simulink model "group2_assignment2_pacemaker"  (R2023b)
settings: Solver=FixedStepAuto  StartTime=0.0  StopTime=10  FixedStep=1e-3  RelTol=1e-3  EnableMultiTasking=on
undefined symbols (not defined in the file): D0, D1, D10, D11, D12, D13, D2, D3, D4, D5, D6, D7, D8, D9, PTA0, PTA1, PTA2, PTB23, PTB9, PTC16, PTC17, PTC2, PTC3, PTC4, PTD0, PTD1, PTD2, PTD3
libraries: frdmk64flib x15, dspstat3 x1
settings Model: SimulationMode=external  ExtModeTrigDuration=5  Creator=stivb  LastModifiedBy=conno
settings OptimizationCC: EnhancedBackFolding=on  PassReuseOutputArgsAs=Individual arguments  ZeroExternalMemoryAtStartup=off  ZeroInternalMemoryAtStartup=off  MaxStackSize=64  OptimizeBlockOrder=speed  DifferentSizesBufferReuse=on  OptimizationCustomize=off  EfficientTunableParamExpr=on
settings DebuggingCC: ParameterTunabilityLossMsg=error
settings HardwareCC: ProdBitPerPointer=32  ProdBitPerSizeT=32  ProdBitPerPtrDiffT=32  ProdLargestAtomicInteger=Long  ProdLargestAtomicFloat=Double  ProdWordSize=32  ProdHWDeviceType=ARM Compatible->ARM Cortex
settings RTWCC: Description=Embedded Coder  SystemTargetFile=ert.tlc  HardwareBoard=NXP FRDM-K64F  TLCOptions="-aInlineSetEventsForThisBaseRateFcn=TLC_FALSE -aSuppressMultiTaskScheduler=TLC_FALSE  -aRateBasedStepFcn=0"  TemplateMakefile=ert_default_tmf  Toolchain=GNU Tools for ARM Embedded Processors
settings CodeAppCC: ForceParamTrailComments=on  IgnoreCustomStorageClasses=off  OperatorAnnotations=on  SimulinkDataObjDesc=on  SFDataObjDesc=on  InsertBlockDesc=on
settings ERTTargetCC: SupportContinuousTime=on  SupportVariableSizeSignals=on  ExtMode=on  ExtModeTransport=4  ExtModeMexFile=sendToCommService  ExtModeMexArgs='group2_assignment2_pacemaker' 0

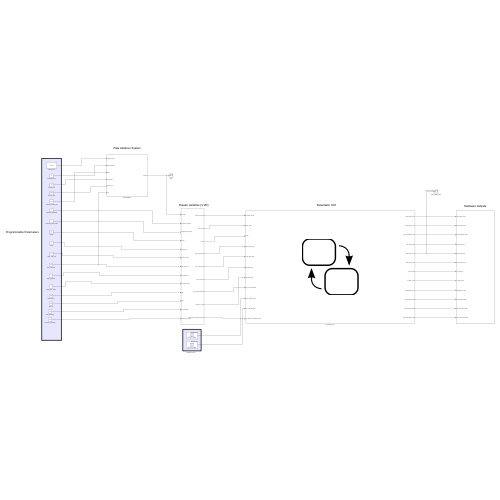
[thumbnail: Simulink's stored preview of the top-level diagram]
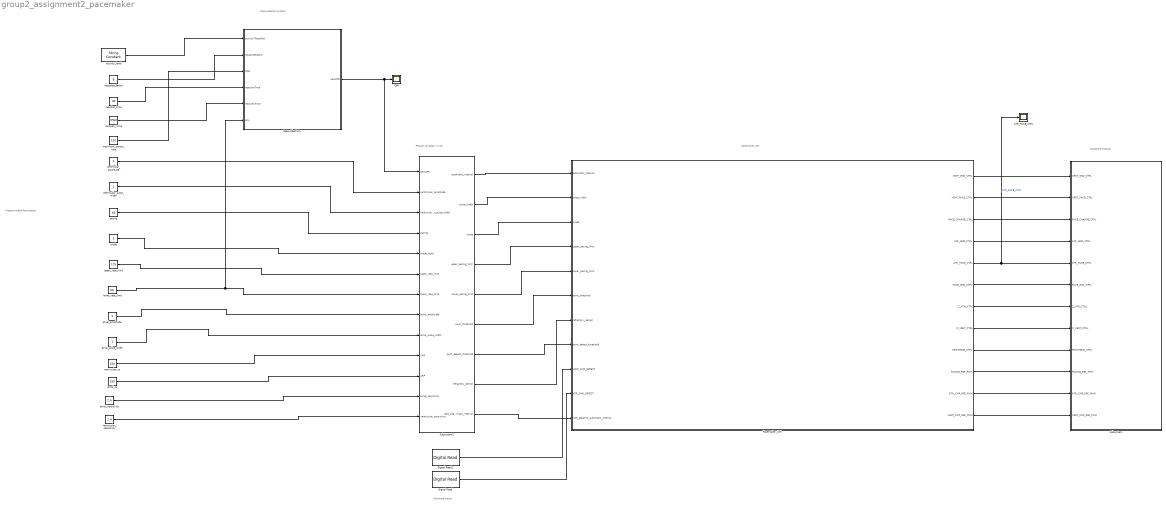
== system group2_assignment2_pacemaker ==
  note: Rate Adaption System
  note: Hardware inputs
  note: Pseudo variables (4 VM)
  note: Programmable Parameters
  note: Pacemaker Unit
  note: Hardware Outputs
  ATR_PACE_CTRL : Scope
  CPR : Scope
  Digital Read : frdmk64flib/Digital Read  Whichpin=PTC16 (D0)  SampleTime=-1
  Digital Read1 : frdmk64flib/Digital Read  Whichpin=PTC17 (D1)  SampleTime=-1
  Pacemaker_Unit : Stateflow chart  TreatAsAtomicUnit=on
      settings: PortSchema="{\"entries\":[{\"content\":{\"sides\":[{\"content\":{\"connectorIds\":[\"In1\",\"In2\",\"In4\",\"In3\",\"In5\",\"In6\",\"In7\",\"In8\",\"In10\",\"In9\",\"In11\"]},\"type\":\"ConnectorPlacement.EquallySpacedRectSide\",\"uuid\":\"c8cba9b3-707c-4f69-ad8c-9d5fbaa12caa\"},{\"content\":{\"connectorIds\":[\"Out1\",\"Out2\",\"Out3\",\"Out4\",\"Out5\",\"Out6\",\"Out7\",\"Out8\",\"Out9\",\"Out10\",\"Out11\",\"Out12\"],\"side\":\"RIGHT\"},\"type\":\"ConnectorPlacement.EquallySpacedRectSide\",\"uuid\":\"918aa1e0-aae1-41d7-a74d-0a72155b1f75\"},{\"content\":{\"side\":\"TOP\"},\"type\":\"ConnectorPlacement.EquallySpacedRectSide\",\"uuid\":\"877803b3-29d8-4e86-807a-7bf9f59cc519\"}]},\"type\":\"ConnectorPlacement.EquallySpacedConnector\",\"uuid\":\"1e148aae-cf3c-4ae1-bc6b-9e679c8c5f2a\"}],\"packageUris\":[\"http://schema.mathworks.com/mf0/Connector/R2020b\"],\"version\":\"1.0\"}"
  Rate Adaptivity : Subsystem
  Subsystem : Subsystem
  Subsystem2 : Subsystem
  activity_level : StringConstant  String="\"V-Low\""
  atrial_amplitude : Constant
  atrial_pulse_width : Constant
  atrial_rp : Constant  Value=150
  atrial_sensitivity : Constant  Value=2.4
  lower_rate_limit : Constant  Value=60
  maximum_sensor_rate : Constant  Value=120
  mode : Constant  Value=3
  pacing : Constant  Value=60
  reaction_time : Constant  Value=30
  recovery_time : Constant  Value=5*60
  response_factor : Constant  Value=8
  upper_rate_limit : Constant  Value=175
  ventricular_amplitude : Constant  Value=4
  ventricular_pulse_width : Constant
  ventricular_rp : Constant  Value=150
  ventricular_sensitivity : Constant  Value=2.4
  wires:
  mode/1 -> Subsystem2/5(mode_input)
  ventricular_amplitude/1 -> Subsystem2/2(ventricular_amplitude)
  atrial_amplitude/1 -> Subsystem2/8(atrial_amplitude)
  atrial_pulse_width/1 -> Subsystem2/9(atrial_pulse_width)
  lower_rate_limit/1 -> Rate Adaptivity/6(LRL), Subsystem2/7(lower_rate_limit)
  upper_rate_limit/1 -> Subsystem2/6(upper_rate_limit)
  ventricular_pulse_width/1 -> Subsystem2/3(ventricular_pulse_width)
  pacing/1 -> Subsystem2/4(pacing)
  Subsystem2/1(automatic_interval) -> Pacemaker_Unit/1(automatic_interval)
  Subsystem2/2(pulse_width) -> Pacemaker_Unit/2(pulse_width)
  Subsystem2/3(mode) -> Pacemaker_Unit/4(mode)
  Subsystem2/4(upper_pacing_limit) -> Pacemaker_Unit/3(upper_pacing_limit)
  Subsystem2/5(lower_pacing_limit) -> Pacemaker_Unit/5(lower_pacing_limit)
  Subsystem2/6(pwm_threshold) -> Pacemaker_Unit/6(pwm_threshold)
  Subsystem2/8(refractory_period) -> Pacemaker_Unit/7(refractory_period)
  Pacemaker_Unit/1(VENT_GND_CTRL) -> Subsystem/1(VENT_GND_CTRL)
  Pacemaker_Unit/2(VENT_PACE_CTRL) -> Subsystem/2(VENT_PACE_CTRL)
  Pacemaker_Unit/3(PACE_CHARGE_CTRL) -> Subsystem/3(PACE_CHARGE_CTRL)
  Pacemaker_Unit/4(ATR_GND_CTRL) -> Subsystem/4(ATR_GND_CTRL)
  Pacemaker_Unit/5(ATR_PACE_CTRL) -> ATR_PACE_CTRL/1, Subsystem/5(ATR_PACE_CTRL)  "ATR_PACE_CTRL"
  Pacemaker_Unit/6(PACE_GND_CTRL) -> Subsystem/6(PACE_GND_CTRL)
  Pacemaker_Unit/7(Z_ATR_CTRL) -> Subsystem/7(Z_ATR_CTRL)
  Pacemaker_Unit/8(Z_VENT_CTRL) -> Subsystem/8(Z_VENT_CTRL)
  Pacemaker_Unit/9(FRONTEND_CTRL) -> Subsystem/9(FRONTEND_CTRL)
  Pacemaker_Unit/10(PACING_REF_PWM) -> Subsystem/10(PACING_REF_PWM)
  ventricular_rp/1 -> Subsystem2/10(VRP)
  atrial_rp/1 -> Subsystem2/11(ARP)
  Pacemaker_Unit/11(ATR_CMP_REF_PWM) -> Subsystem/11(ATR_CMP_REF_PWM)
  Digital Read/1 -> Pacemaker_Unit/9(ATR_CMP_DETECT)
  Digital Read1/1 -> Pacemaker_Unit/10(VENT_CMP_DETECT)
  atrial_sensitivity/1 -> Subsystem2/12(atrial_sensitivity)
  ventricular_sensitivity/1 -> Subsystem2/13(ventricular_sensitivity)
  Subsystem2/7(pwm_detect_threshold) -> Pacemaker_Unit/8(pwm_detect_threshold)
  Pacemaker_Unit/12(VENT_CMP_REF_PWM) -> Subsystem/12(VENT_CMP_REF_PWM)
  Subsystem2/9(rate_adaptive_automatic_interval) -> Pacemaker_Unit/11(rate_adaptive_automatic_interval)
  activity_level/1 -> Rate Adaptivity/1(activityThreshold)
  response_factor/1 -> Rate Adaptivity/2(responseFactor)
  maximum_sensor_rate/1 -> Rate Adaptivity/3(MSR)
  reaction_time/1 -> Rate Adaptivity/4(reactionTime)
  recovery_time/1 -> Rate Adaptivity/5(recoveryTime)
  Rate Adaptivity/1(newCPR) -> CPR/1, Subsystem2/1(newCPR)

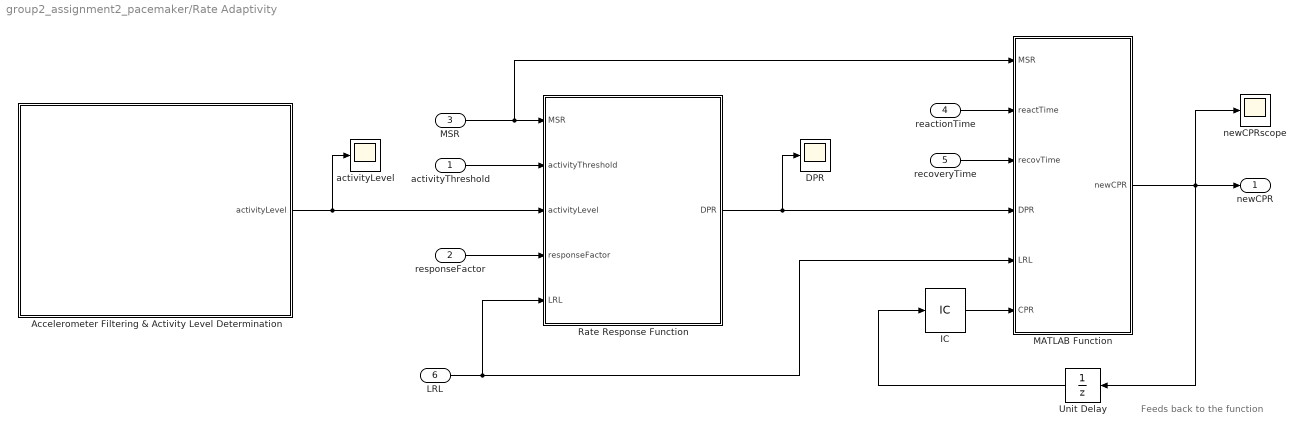
== system group2_assignment2_pacemaker/Rate Adaptivity ==
  note: Feeds back to the function
  activityThreshold : Inport
  responseFactor : Inport  Port=2
  MSR : Inport  Port=3
  reactionTime : Inport  Port=4
  recoveryTime : Inport  Port=5
  LRL : Inport  Port=6
  Accelerometer Filtering & Activity Level Determination : Subsystem
  DPR : Scope
  IC : InitialCondition  Value=80
  MATLAB Function : MATLAB Function  TreatAsAtomicUnit=on
  Rate Response Function : MATLAB Function  TreatAsAtomicUnit=on
  Unit Delay : UnitDelay  SampleTime=-1  HasFrameUpgradeWarning=on
  activityLevel : Scope
  newCPRscope : Scope
  newCPR : Outport
  wires:
  LRL/1 -> MATLAB Function/5(LRL), Rate Response Function/5(LRL)
  activityThreshold/1 -> Rate Response Function/2(activityThreshold)
  MSR/1 -> MATLAB Function/1(MSR), Rate Response Function/1(MSR)
  responseFactor/1 -> Rate Response Function/4(responseFactor)
  recoveryTime/1 -> MATLAB Function/3(recovTime)
  MATLAB Function/1(newCPR) -> Unit Delay/1, newCPR/1, newCPRscope/1
  reactionTime/1 -> MATLAB Function/2(reactTime)
  Rate Response Function/1(DPR) -> MATLAB Function/4(DPR), DPR/1
  Unit Delay/1 -> IC/1
  IC/1 -> MATLAB Function/6(CPR)
  Accelerometer Filtering & Activity Level Determination/1(activityLevel) -> Rate Response Function/3(activityLevel), activityLevel/1

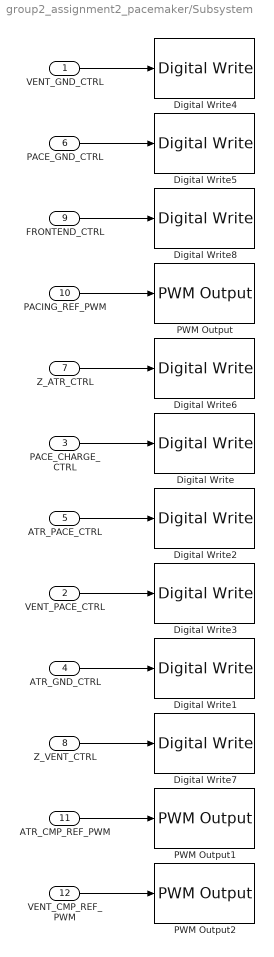
== system group2_assignment2_pacemaker/Subsystem ==
  VENT_GND_CTRL : Inport
  VENT_PACE_CTRL : Inport  Port=2
  PACE_CHARGE_CTRL : Inport  Port=3
  ATR_GND_CTRL : Inport  Port=4
  ATR_PACE_CTRL : Inport  Port=5
  PACE_GND_CTRL : Inport  Port=6
  Z_ATR_CTRL : Inport  Port=7
  Z_VENT_CTRL : Inport  Port=8
  FRONTEND_CTRL : Inport  Port=9
  PACING_REF_PWM : Inport  Port=10
  ATR_CMP_REF_PWM : Inport  Port=11
  VENT_CMP_REF_PWM : Inport  Port=12
  Digital Write : frdmk64flib/Digital Write  Whichpin=PTB9 (D2)
  Digital Write1 : frdmk64flib/Digital Write  Whichpin=PTD2 (D11)
  Digital Write2 : frdmk64flib/Digital Write  Whichpin=PTA0 (D8)
  Digital Write3 : frdmk64flib/Digital Write  Whichpin=PTC4 (D9)
  Digital Write4 : frdmk64flib/Digital Write  Whichpin=PTD3 (D12)
  Digital Write5 : frdmk64flib/Digital Write  Whichpin=PTD0 (D10)
  Digital Write6 : frdmk64flib/Digital Write  Whichpin=PTB23 (D4)
  Digital Write7 : frdmk64flib/Digital Write  Whichpin=PTC3 (D7)
  Digital Write8 : frdmk64flib/Digital Write  Whichpin=PTD1 (D13)
  PWM Output : frdmk64flib/PWM Output  Whichpin=PTA2 (D5)  InitialFrequency=2000  InitialDutyCycle=0
  PWM Output1 : frdmk64flib/PWM Output  Whichpin=PTC2 (D6)  InitialFrequency=2000  InitialDutyCycle=0
  PWM Output2 : frdmk64flib/PWM Output  Whichpin=PTA1 (D3)  InitialFrequency=2000  InitialDutyCycle=0
  wires:
  Z_ATR_CTRL/1 -> Digital Write6/1
  VENT_PACE_CTRL/1 -> Digital Write3/1
  FRONTEND_CTRL/1 -> Digital Write8/1
  PACING_REF_PWM/1 -> PWM Output/1
  ATR_PACE_CTRL/1 -> Digital Write2/1
  Z_VENT_CTRL/1 -> Digital Write7/1
  VENT_GND_CTRL/1 -> Digital Write4/1
  PACE_CHARGE_CTRL/1 -> Digital Write/1
  ATR_GND_CTRL/1 -> Digital Write1/1
  PACE_GND_CTRL/1 -> Digital Write5/1
  ATR_CMP_REF_PWM/1 -> PWM Output1/1
  VENT_CMP_REF_PWM/1 -> PWM Output2/1

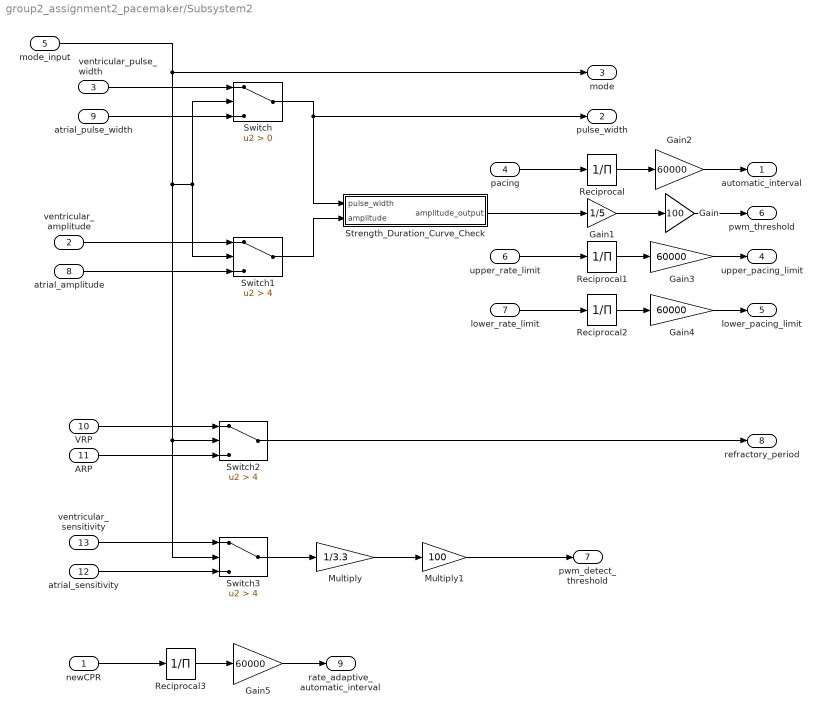
== system group2_assignment2_pacemaker/Subsystem2 ==
  newCPR : Inport
  ventricular_amplitude : Inport  Port=2
  ventricular_pulse_width : Inport  Port=3
  pacing : Inport  Port=4
  mode_input : Inport  Port=5
  upper_rate_limit : Inport  Port=6
  lower_rate_limit : Inport  Port=7
  atrial_amplitude : Inport  Port=8
  atrial_pulse_width : Inport  Port=9
  VRP : Inport  Port=10
  ARP : Inport  Port=11
  atrial_sensitivity : Inport  Port=12
  ventricular_sensitivity : Inport  Port=13
  Gain : Gain  Gain=100
  Gain1 : Gain  Gain=1/5
  Gain{2..5} (4 alike) : Gain  Gain=60000
  Multiply : Gain  Gain=1/3.3
  Multiply1 : Gain  Gain=100
  Reciprocal{,1..3} (4 alike) : Product  Inputs=/
  Strength_Duration_Curve_Check : Stateflow chart  TreatAsAtomicUnit=on
  Switch : Switch  Criteria=u2 > Threshold  SaturateOnIntegerOverflow=off  InputSameDT=off
  Switch1 : Switch  Criteria=u2 > Threshold  Threshold=4  SaturateOnIntegerOverflow=off  InputSameDT=off
  Switch2 : Switch  Criteria=u2 > Threshold  Threshold=4  SaturateOnIntegerOverflow=off  InputSameDT=off
  Switch3 : Switch  Criteria=u2 > Threshold  Threshold=4  SaturateOnIntegerOverflow=off  InputSameDT=off
  automatic_interval : Outport
  pulse_width : Outport  Port=2
  mode : Outport  Port=3
  upper_pacing_limit : Outport  Port=4
  lower_pacing_limit : Outport  Port=5
  pwm_threshold : Outport  Port=6
  pwm_detect_threshold : Outport  Port=7
  refractory_period : Outport  Port=8
  rate_adaptive_automatic_interval : Outport  Port=9
  wires:
  Gain1/1 -> Gain/1
  pacing/1 -> Reciprocal/1
  Reciprocal1/1 -> Gain3/1
  upper_rate_limit/1 -> Reciprocal1/1
  Reciprocal/1 -> Gain2/1
  Gain2/1 -> automatic_interval/1
  Gain/1 -> pwm_threshold/1
  Gain3/1 -> upper_pacing_limit/1
  Strength_Duration_Curve_Check/1(amplitude_output) -> Gain1/1
  Reciprocal2/1 -> Gain4/1
  lower_rate_limit/1 -> Reciprocal2/1
  Gain4/1 -> lower_pacing_limit/1
  Switch1/1 -> Strength_Duration_Curve_Check/2(amplitude)
  Switch/1 -> Strength_Duration_Curve_Check/1(pulse_width), pulse_width/1
  Switch2/1 -> refractory_period/1
  VRP/1 -> Switch2/1
  ARP/1 -> Switch2/3
  ventricular_amplitude/1 -> Switch1/1
  ventricular_pulse_width/1 -> Switch/1
  atrial_pulse_width/1 -> Switch/3
  atrial_amplitude/1 -> Switch1/3
  mode_input/1 -> Switch3/2, Switch2/2, Switch1/2, Switch/2, mode/1
  atrial_sensitivity/1 -> Switch3/3
  ventricular_sensitivity/1 -> Switch3/1
  Switch3/1 -> Multiply/1
  Multiply/1 -> Multiply1/1
  Multiply1/1 -> pwm_detect_threshold/1
  Gain5/1 -> rate_adaptive_automatic_interval/1
  Reciprocal3/1 -> Gain5/1
  newCPR/1 -> Reciprocal3/1

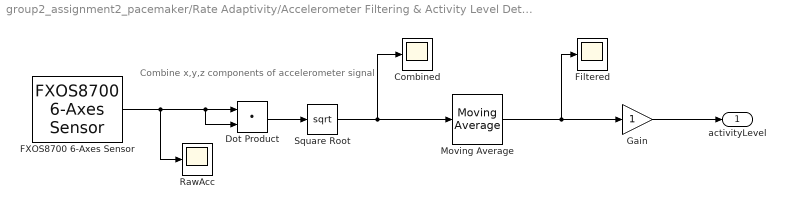
== system group2_assignment2_pacemaker/Rate Adaptivity/Accelerometer Filtering & Activity Level Determination ==
  note: Combine x,y,z components of accelerometer signal
  Combined : Scope
  Dot Product : DotProduct  OutDataTypeStr=Inherit: Inherit via internal rule
  FXOS8700 6-Axes Sensor : frdmk64flib/FXOS8700 6-Axes Sensor  Activesensor=Accelerometer only  ODR=800Hz  HybridODR=400Hz  Accelfullrange=-4g to +4g  SampleTime=-1
  Filtered : Scope
  Gain : Gain
  Moving Average : dspstat3/Moving Average  Method=Sliding window  ForgettingFactorPort=off  SpecifyWindowLength=on  WindowLength=4  OverlapLength=3  AllowArbitraryInputLength=off  ForgettingFactor=0.9  SimulateUsing=Code generation
  RawAcc : Scope
  Square Root : Sqrt
  activityLevel : Outport
  wires:
  Moving Average/1 -> Filtered/1, Gain/1
  Square Root/1 -> Moving Average/1, Combined/1
  Dot Product/1 -> Square Root/1
  FXOS8700 6-Axes Sensor/1 -> Dot Product/1, Dot Product/2, RawAcc/1
  Gain/1 -> activityLevel/1

== stateflow chart group2_assignment2_pacemaker/Pacemaker_Unit ==
  state VOO
    state Charge_C22_Discharge_C21
      entry:
      %Charge C22
      VENT_PACE_CTRL = 0;
      PACE_CHARGE_CTRL = 1;
      %Discharge C21
      VENT_GND_CTRL= 1;
    state ChargeC21_and_DischargeC22
      %Creates the leading edge and sends pulse for X amount of time
      entry:
      PACE_CHARGE_CTRL = 0;
      VENT_GND_CTRL = 0;
      VENT_PACE_CTRL = 1;
      %Recharge pulse is the current in the opposite direction due to C21
    (default) -> VOO.Charge_C22_Discharge_C21
    VOO.Charge_C22_Discharge_C21 -> VOO.ChargeC21_and_DischargeC22 : after(automatic_interval-pulse_width, msec)
    VOO.ChargeC21_and_DischargeC22 -> VOO.Charge_C22_Discharge_C21 : after(pulse_width, msec)
  state VVI
    note: Safe start entry; since hysteresis pacing allows for waiting a period of time longer than the refractory period, we are okay with waiting a refractory period of time before we start pacing. This also ensures that the capacitors are appropriately charged to allow for proper pacing.
    state Refractory_and_charging_ventricle
      entry:
      %Charge C22
      VENT_PACE_CTRL = 0;
      PACE_CHARGE_CTRL = 1;
      %Discharge C21
      VENT_GND_CTRL= 1;
      % Setup sensing pins
      VENT_CMP_REF_PWM = pwm_detect_threshold;
    note: Detected a pace, so go back to refractory state to wait
        | the appropriate refractory time interval
    state Sensing_ventricle
      entry:
      FRONTEND_CTRL = 1;
    state Pacing_ventricle
      entry:
      PACE_CHARGE_CTRL = 0;
      VENT_PACE_CTRL = 1;
      VENT_GND_CTRL = 0;
    (default) -> VVI.Refractory_and_charging_ventricle
    VVI.Refractory_and_charging_ventricle -> VVI.Sensing_ventricle : after(refractory_period, msec)
    VVI.Sensing_ventricle -> VVI.Refractory_and_charging_ventricle [order 1] : [VENT_CMP_DETECT == true]
    VVI.Pacing_ventricle -> VVI.Refractory_and_charging_ventricle : after(pulse_width, msec)
    VVI.Sensing_ventricle -> VVI.Pacing_ventricle [order 2] : after(automatic_interval - refractory_period - pulse_width, msec)
  state Ventricular_Safe_State
    entry: %Safe State
    ATR_PACE_CTRL = 0;
    VENT_PACE_CTRL=0;
    PACING_REF_PWM = pwm_threshold;
    PACE_CHARGE_CTRL=0;
    PACE_GND_CTRL = 1;
    VENT_PACE_CTRL=0;
    Z_ATR_CTRL=0;
    Z_VENT_CTRL=0;
    ATR_PACE_CTRL=0;
    ATR_GND_CTRL=0;
    VENT_GND_CTRL=1;
    FRONTEND_CTRL=0;
  state VOOR
    state Charge_C22_Discharge_C21
      entry:
      %Charge C22
      VENT_PACE_CTRL = 0;
      PACE_CHARGE_CTRL = 1;
      %Discharge C21
      VENT_GND_CTRL= 1;
    state ChargeC21_and_DischargeC22
      %Creates the leading edge and sends pulse for X amount of time
      entry:
      PACE_CHARGE_CTRL = 0;
      VENT_GND_CTRL = 0;
      VENT_PACE_CTRL = 1;
      %Recharge pulse is the current in the opposite direction due to C21
    (default) -> VOOR.Charge_C22_Discharge_C21
    VOOR.Charge_C22_Discharge_C21 -> VOOR.ChargeC21_and_DischargeC22 : after(rate_adaptive_automatic_interval-pulse_width, msec)
    VOOR.ChargeC21_and_DischargeC22 -> VOOR.Charge_C22_Discharge_C21 : after(pulse_width, msec)
  state VVIR
    note: Safe start entry; since hysteresis pacing allows for waiting a period of time longer than the refractory period, we are okay with waiting a refractory period of time before we start pacing. This also ensures that the capacitors are appropriately charged to allow for proper pacing.
    state Refractory_and_charging_ventricle
      entry:
      %Charge C22
      VENT_PACE_CTRL = 0;
      PACE_CHARGE_CTRL = 1;
      %Discharge C21
      VENT_GND_CTRL= 1;
      % Setup sensing pins
      VENT_CMP_REF_PWM = pwm_detect_threshold;
    note: Detected a pace, so go back to refractory state to wait
        | the appropriate refractory time interval
    state Sensing_ventricle
      entry:
      FRONTEND_CTRL = 1;
    state Pacing_ventricle
      entry:
      PACE_CHARGE_CTRL = 0;
      VENT_PACE_CTRL = 1;
      VENT_GND_CTRL = 0;
    (default) -> VVIR.Refractory_and_charging_ventricle
    VVIR.Refractory_and_charging_ventricle -> VVIR.Sensing_ventricle : after(refractory_period, msec)
    VVIR.Sensing_ventricle -> VVIR.Refractory_and_charging_ventricle [order 1] : [VENT_CMP_DETECT == true]
    VVIR.Pacing_ventricle -> VVIR.Refractory_and_charging_ventricle : after(pulse_width, msec)
    VVIR.Sensing_ventricle -> VVIR.Pacing_ventricle [order 2] : after(rate_adaptive_automatic_interval - refractory_period - pulse_width, msec)
  state Mode_Selection
  state AAIR
    note: Safe start entry; since hysteresis pacing allows for waiting a period of time longer than the refractory period, we are okay with waiting a refractory period of time before we start pacing. This also ensures that the capacitors are appropriately charged to allow for proper pacing.
    state Refractory_and_charging_atrial
      entry:
      %Charge C22
      ATR_PACE_CTRL = 0;
      PACE_CHARGE_CTRL = 1;
      %Discharge C21
      ATR_GND_CTRL= 1;
      % Setup sensing pins
      ATR_CMP_REF_PWM = pwm_detect_threshold;
    note: Detected a pace, so go back to refractory state to wait
        | the appropriate refractory time interval
    state Sensing_atrial
      entry:
      FRONTEND_CTRL = 1;
    state Pacing_atrial
      entry:
      PACE_CHARGE_CTRL = 0;
      ATR_PACE_CTRL = 1;
      ATR_GND_CTRL = 0;
    (default) -> AAIR.Refractory_and_charging_atrial
    AAIR.Refractory_and_charging_atrial -> AAIR.Sensing_atrial : after(refractory_period, msec)
    AAIR.Sensing_atrial -> AAIR.Refractory_and_charging_atrial [order 1] : [ATR_CMP_DETECT == true]
    AAIR.Pacing_atrial -> AAIR.Refractory_and_charging_atrial : after(pulse_width, msec)
    AAIR.Sensing_atrial -> AAIR.Pacing_atrial [order 2] : after(rate_adaptive_automatic_interval - refractory_period - pulse_width, msec)
  state Atrial_Safe_State
    entry: %Safe State
    ATR_PACE_CTRL = 0;
    VENT_PACE_CTRL=0;
    PACING_REF_PWM = pwm_threshold;
    PACE_CHARGE_CTRL=0;
    PACE_GND_CTRL = 1;
    VENT_PACE_CTRL=0;
    Z_ATR_CTRL=0;
    Z_VENT_CTRL=0;
    ATR_PACE_CTRL=0;
    ATR_GND_CTRL=1;
    VENT_GND_CTRL=0;
    FRONTEND_CTRL=0;
  state AOOR
    state Charge_C22_Discharge_C21
      entry:
      %Charge C22
      ATR_PACE_CTRL = 0;
      PACE_CHARGE_CTRL = 1;
      %Discharge C21
      ATR_GND_CTRL= 1;
    state ChargeC21_and_DischargeC22
      %Creates the leading edge and sends pulse for X amount of time
      entry:
      PACE_CHARGE_CTRL = 0;
      ATR_PACE_CTRL = 1;
      ATR_GND_CTRL = 0;
    (default) -> AOOR.Charge_C22_Discharge_C21
    AOOR.Charge_C22_Discharge_C21 -> AOOR.ChargeC21_and_DischargeC22 : after(rate_adaptive_automatic_interval-pulse_width, msec)
    AOOR.ChargeC21_and_DischargeC22 -> AOOR.Charge_C22_Discharge_C21 : after(pulse_width, msec)
  state AAI
    note: Safe start entry; since hysteresis pacing allows for waiting a period of time longer than the refractory period, we are okay with waiting a refractory period of time before we start pacing. This also ensures that the capacitors are appropriately charged to allow for proper pacing.
    state Refractory_and_charging_atrial
      entry:
      %Charge C22
      ATR_PACE_CTRL = 0;
      PACE_CHARGE_CTRL = 1;
      %Discharge C21
      ATR_GND_CTRL= 1;
      % Setup sensing pins
      ATR_CMP_REF_PWM = pwm_detect_threshold;
    note: Detected a pace, so go back to refractory state to wait
        | the appropriate refractory time interval
    state Sensing_atrial
      entry:
      FRONTEND_CTRL = 1;
    state Pacing_atrial
      entry:
      PACE_CHARGE_CTRL = 0;
      ATR_PACE_CTRL = 1;
      ATR_GND_CTRL = 0;
    (default) -> AAI.Refractory_and_charging_atrial
    AAI.Refractory_and_charging_atrial -> AAI.Sensing_atrial : after(refractory_period, msec)
    AAI.Sensing_atrial -> AAI.Refractory_and_charging_atrial [order 1] : [ATR_CMP_DETECT == true]
    AAI.Pacing_atrial -> AAI.Refractory_and_charging_atrial : after(pulse_width, msec)
    AAI.Sensing_atrial -> AAI.Pacing_atrial [order 2] : after(automatic_interval - refractory_period - pulse_width, msec)
  state AOO
    state Charge_C22_Discharge_C21
      entry:
      %Charge C22
      ATR_PACE_CTRL = 0;
      PACE_CHARGE_CTRL = 1;
      %Discharge C21
      ATR_GND_CTRL= 1;
    state ChargeC21_and_DischargeC22
      %Creates the leading edge and sends pulse for X amount of time
      entry:
      PACE_CHARGE_CTRL = 0;
      ATR_PACE_CTRL = 1;
      ATR_GND_CTRL = 0;
    (default) -> AOO.Charge_C22_Discharge_C21
    AOO.Charge_C22_Discharge_C21 -> AOO.ChargeC21_and_DischargeC22 : after(automatic_interval-pulse_width, msec)
    AOO.ChargeC21_and_DischargeC22 -> AOO.Charge_C22_Discharge_C21 : after(pulse_width, msec)
  (junction 25) -> VOO [order 1] : [mode == 5]
  (junction 25) -> VVI [order 2] : [mode == 6]
  Ventricular_Safe_State -> (junction 25)
  (junction 25) -> VOOR [order 3] : [mode == 7]
  (junction 25) -> VVIR [order 4] : [mode == 8]
  Mode_Selection -> Ventricular_Safe_State [order 1] : [mode>4]
  (default) -> Mode_Selection
  Mode_Selection -> Atrial_Safe_State [order 2] : [mode <= 4]
  (junction 60) -> AAIR [order 4] : [mode == 4]
  (junction 60) -> AOOR [order 3] : [mode == 3]
  Atrial_Safe_State -> (junction 60)
  (junction 60) -> AAI [order 2] : [mode == 2]
  (junction 60) -> AOO [order 1] : [mode == 1]
  data: automatic_interval input; pulse_width input; upper_pacing_limit input; mode input; lower_pacing_limit input; pwm_threshold input; refractory_period input; VENT_GND_CTRL output; VENT_PACE_CTRL output; PACE_CHARGE_CTRL output; ATR_GND_CTRL output; ATR_PACE_CTRL output; PACE_GND_CTRL output; Z_ATR_CTRL output; Z_VENT_CTRL output; FRONTEND_CTRL output; PACING_REF_PWM output; pwm_detect_threshold input; ATR_CMP_DETECT input; ATR_CMP_REF_PWM output; VENT_CMP_DETECT input; VENT_CMP_REF_PWM output; rate_adaptive_automatic_interval input

== matlab function group2_assignment2_pacemaker/Rate Adaptivity/MATLAB Function ==
  data: MSR input; newCPR output; reactTime input; recovTime input; DPR input; LRL input; CPR input
    function newCPR = timing(MSR, reactTime, recovTime, DPR, LRL, CPR)
if (CPR < DPR) && (CPR < MSR) % Increase Rate

    % Current Time based on Current Pace
    currTime = -log(1 - (LRL - CPR)/(LRL - MSR))*(reactTime/11 - 2/11);
    % Increase current time by 1ms
    currTime = currTime + 0.001;
    % New Pace Rate after 1ms increase
    newCPR = (1-exp(-11*currTime/(reactTime-2)))*(MSR-LRL) + LRL;

elseif (CPR > DPR) && (CPR > LRL) % Decrease Rate

    %Current Time based on Current Pace
    currTime = -log((LRL - CPR)/(LRL - MSR))*(recovTime/11 - 3/11);
    % Increase time by 1ms
    currTime = currTime + 0.001;
    %New Pace Rate after 1ms increase
    newCPR = (exp(-11*currTime/(recovTime-3)))*(MSR-LRL) + LRL;
      
else 
    newCPR = CPR; 

end
end

== stateflow chart group2_assignment2_pacemaker/Subsystem2/Strength_Duration_Curve_Check ==
  state amplitude_too_low_short_duration
    entry:
    amplitude_output = 4;
  state appropriate_amplitude1
    entry:
    amplitude_output = amplitude;
  state amplitude_too_high_short_duration
    entry:
    amplitude_output = 5;
  state Initalize
  state amplitude_too_low
    entry:
    amplitude_output = 1.6;
  state appropriate_amplitude
    entry:
    amplitude_output = amplitude;
  state amplitude_too_high
    entry:
    amplitude_output = 5;
  (junction 14) -> amplitude_too_low_short_duration [order 2] : [amplitude<4]
  (junction 30) -> appropriate_amplitude1 [order 1] : [amplitude<=5]
  Initalize -> (junction 14) [order 1] : [pulse_width<0.5]
  (junction 14) -> (junction 30) [order 1] : [amplitude>=4]
  (junction 30) -> amplitude_too_high_short_duration [order 2] : [amplitude>5]
  (default) -> Initalize
  Initalize -> (junction 8) [order 2] : [pulse_width>=0.5]
  (junction 8) -> amplitude_too_low [order 2] : [amplitude<1.6]
  (junction 8) -> (junction 22) [order 1] : [amplitude>=1.6]
  (junction 22) -> appropriate_amplitude [order 1] : [amplitude<=5]
  (junction 22) -> amplitude_too_high [order 2] : [amplitude>5]
  data: pulse_width input; amplitude input; amplitude_output output

== matlab function group2_assignment2_pacemaker/Rate Adaptivity/Rate Response Function ==
  data: MSR input; activityThreshold input; DPR output; activityLevel input; responseFactor input; LRL input
function DPR  = fcn(MSR, activityThreshold, activityLevel, responseFactor, LRL)

% total range of change of acceleration 
ATMax = sqrt(4^2+4^2+4^2)-1; 

% since the accelerameter record the gravity (1g), 1g is removed to ensure when the pacemaker is static, there is no extra pacing 
activityThresholdLevels = {'V-Low', 'Low', 'Med-Low', 'Med', 'Med-High', 'High', 'V-High'}; %possible activity level string inputs

activityThresholdRange = [0.05*ATMax+1, 0.15*ATMax+1, 0.30*ATMax+1, 0.45*ATMax+1, 0.60*ATMax+1, 0.75*ATMax+1, 0.90*ATMax+1]; 
%take percentage of a maximum activity level, plus on to ensure the threshold is higher than defaul 1g (default acceleration reading

activityThresholdNum = activityThresholdRange(find(strcmp(activityThresholdLevels, char(activityThreshold)))); 
%map the string level of activity levels to a number value


if(activityLevel <= activityThresholdNum(1)) %doesn't meet the activity level threshold
    DPR = LRL;

elseif(activityLevel > activityThresholdNum(1) && activityLevel < sqrt(48))  % when the activity level is between threshold and max activity
    DPR = (1-exp((-(1/(sqrt(48)-activityLevel)*responseFactor*(activityLevel-activityThresholdNum(1))))))*(MSR-LRL)+LRL;

else
    DPR = MSR; %set to max sensor rate if activity level is greater than max activity

end
end
